simulink model "imp_test"  (R2022b)
settings: Solver=FixedStepDiscrete  StartTime=0.0  StopTime=10.0  FixedStep=0.001  RelTol=1e-3
settings Model: Creator=brl-pc3-ubuntu  LastModifiedBy=brl-pc3-ubuntu

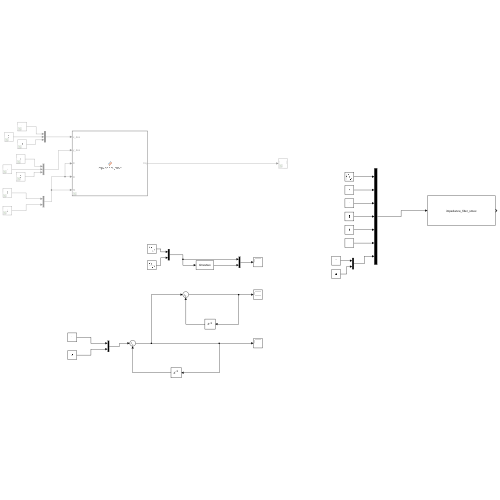
[thumbnail: Simulink's stored preview of the top-level diagram]
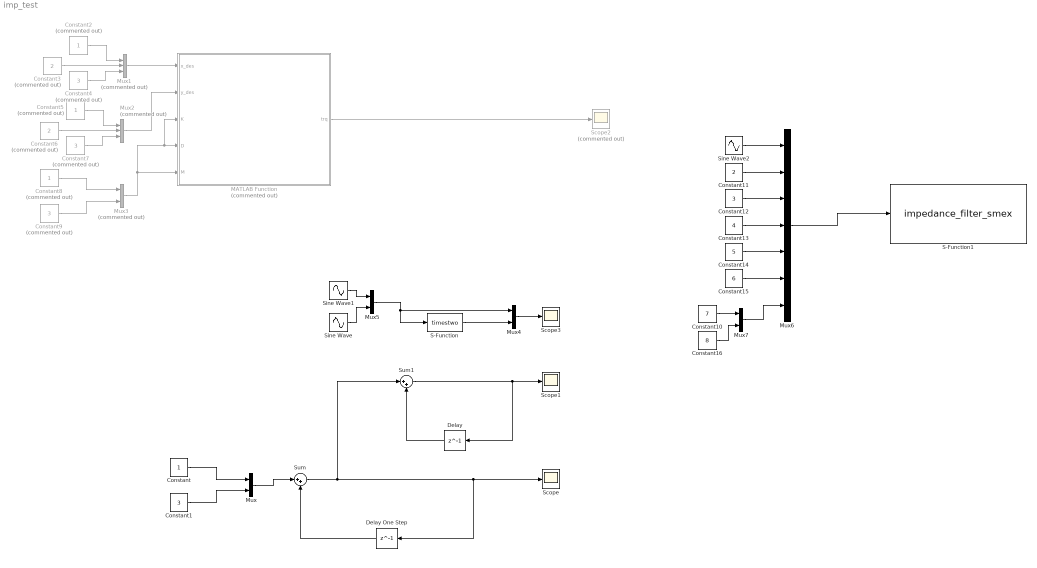
== system imp_test ==
  Constant : Constant
  Constant1 : Constant  Value=3
  Constant10 : Constant  Value=7
  Constant11 : Constant  Value=2
  Constant12 : Constant  Value=3
  Constant13 : Constant  Value=4
  Constant14 : Constant  Value=5
  Constant15 : Constant  Value=6
  Constant16 : Constant  Value=8
  Constant2 : Constant  Commented=on
  Constant3 : Constant  Commented=on  Value=2
  Constant4 : Constant  Commented=on  Value=3
  Constant5 : Constant  Commented=on
  Constant6 : Constant  Commented=on  Value=2
  Constant7 : Constant  Commented=on  Value=3
  Constant8 : Constant  Commented=on
  Constant9 : Constant  Commented=on  Value=3
  Delay : Delay  DelayLength=1
  Delay One Step : Delay  DelayLength=1
  MATLAB Function : MATLAB Function  Commented=on  TreatAsAtomicUnit=on
  Mux{,4..5,7} (4 alike) : Mux  Inputs=2
  Mux1 : Mux  Commented=on  Inputs=3
  Mux2 : Mux  Commented=on  Inputs=3
  Mux3 : Mux  Commented=on  Inputs=2
  Mux6 : Mux  Inputs=7
  S-Function : S-Function  FunctionName=timestwo  SFunctionDeploymentMode=off  EnableBusSupport=off
  S-Function1 : S-Function  FunctionName=impedance_filter_smex  SFunctionDeploymentMode=off  EnableBusSupport=off
  Scope : Scope
  Scope1 : Scope
  Scope2 : Scope  Commented=on
  Scope3 : Scope
  Sine Wave : Sin  SampleTime=0
  Sine Wave1 : Sin  Bias=10  SampleTime=0
  Sine Wave2 : Sin  Bias=10  SampleTime=0
  Sum : Sum  Inputs=|++
  Sum1 : Sum  Inputs=|++
  wires:
  Constant/1 -> Mux/1
  Delay One Step/1 -> Sum/2
  Sum/1 -> Delay One Step/1, Scope/1, Sum1/1
  Sum1/1 -> Delay/1, Scope1/1
  Delay/1 -> Sum1/2
  Constant1/1 -> Mux/2
  Mux/1 -> Sum/1
  Mux1/1 -> MATLAB Function/1(x_des)
  Constant2/1 -> Mux1/1
  Constant3/1 -> Mux1/2
  Constant4/1 -> Mux1/3
  Constant7/1 -> Mux2/3
  Mux2/1 -> MATLAB Function/2(y_des)
  Constant6/1 -> Mux2/2
  Constant5/1 -> Mux2/1
  Constant9/1 -> Mux3/2
  Constant8/1 -> Mux3/1
  Mux3/1 -> MATLAB Function/5(M), MATLAB Function/4(D), MATLAB Function/3(K)
  MATLAB Function/1(trq) -> Scope2/1
  Sine Wave/1 -> Mux5/2
  S-Function/1 -> Mux4/2
  Mux4/1 -> Scope3/1
  Sine Wave1/1 -> Mux5/1
  Mux5/1 -> Mux4/1, S-Function/1
  Mux6/1 -> S-Function1/1
  Sine Wave2/1 -> Mux6/1
  Constant15/1 -> Mux6/6
  Constant14/1 -> Mux6/5
  Constant13/1 -> Mux6/4
  Constant12/1 -> Mux6/3
  Constant11/1 -> Mux6/2
  Constant10/1 -> Mux7/1
  Mux7/1 -> Mux6/7
  Constant16/1 -> Mux7/2

== matlab function imp_test/MATLAB Function ==
  data: x_des input; trq output; y_des input; K input; D input; M input
function trq = impedance_filter(x_des, y_des, K, D, M)
trq = impedance_filter_mex(x_des, y_des, K, D, M);
